simulink model "torqueBalancing"  (Simulink 8.6)
settings: Solver=FixedStepDiscrete  StartTime=0.0  StopTime=simulationTime  FixedStep=Ts  RelTol=1e-3
InitFcn:
  | initTorqueBalancing;
undefined symbols (not defined in the file): bVectorConstraints, ConstraintsMatrix, DEMO_MOVEMENTS, DiscIntNeverNeededParam, gain, impedencesSat, LEFT_RIGHT_FOOT_IN_CONTACT, localName, ON_GAZEBO, reg, ROBOT_DOF, ROBOT_DOF_FOR_SIMULINK, robotName, sat, sm, SMOOTH_DES_COM, SMOOTH_DES_Q, Ts, USE_QP_SOLVER, USE_SM
libraries: WBCLibrary x61, simulink x3
settings Model: Creator=daniele  LastModifiedBy=DanielePucci
settings DataIOCC: SignalLoggingSaveFormat=Dataset
settings DebuggingCC: FcnCallInpInsideContextMsg=EnableAllAsWarning
settings SFSimCC: SimParseCustomCode=off
settings ConfigComp: CovSFcnEnable=off

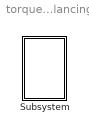
== system torqueBalancing ==
  Subsystem : Subsystem  mask{robotName=robotName, Ts=Ts, localName=localName}
      mask prompts: robotName "robot name"; localName "module name"

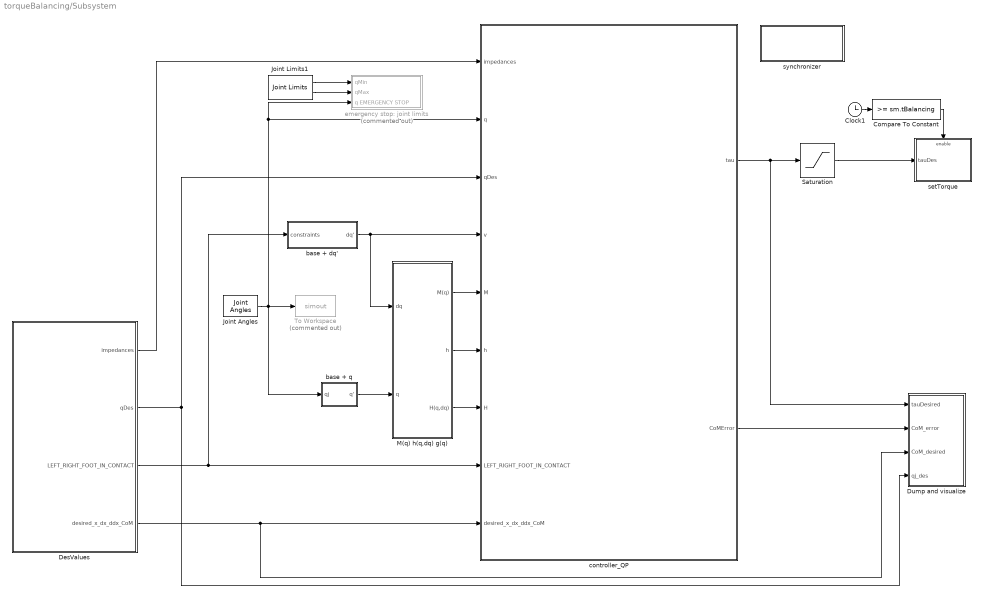
== system torqueBalancing/Subsystem ==
  Clock1 : Clock
  Compare To Constant : simulink/Logic and Bit Operations/Compare To Constant  relop=>=  const=sm.tBalancing  OutDataTypeStr=boolean
  DesValues : Subsystem  Priority=-10
  Dump and visualize : Subsystem
  Joint Angles : WBCLibrary/wholeBodyStates/Joint Angles  robotName=robotName  localName=localName
  Joint Limits1 : WBCLibrary/wholeBodyModel/Joint Limits  robotName=robotName  localName=localName
  M(q) h(q,dq) g(q) : Subsystem
  Saturation : Saturate  UpperLimit=sat.torque  LowerLimit=-sat.torque
  To Workspace : ToWorkspace  Commented=on  VariableName=simout  SaveFormat=Timeseries  SampleTime=-1
  base + dq' : Subsystem
  base + q : Subsystem
  controller_QP : Subsystem
  emergency stop: joint limits : Subsystem  Commented=on
  setTorque : Subsystem
  synchronizer : Subsystem
      mask Display: disp('SYNCHRONIZER')
  wires:
  base + q/1(q') -> M(q) h(q,dq) g(q)/2(q)
  base + dq'/1(dq') -> controller_QP/4(v), M(q) h(q,dq) g(q)/1(dq)
  M(q) h(q,dq) g(q)/1(M(q)) -> controller_QP/5(M)
  Joint Limits1/1 -> emergency stop: joint limits/1(qMin)
  Joint Limits1/2 -> emergency stop: joint limits/2(qMax)
  Joint Angles/1 -> To Workspace/1, base + q/1(qj), emergency stop: joint limits/3(q EMERGENCY STOP), controller_QP/2(q)
  M(q) h(q,dq) g(q)/2(h) -> controller_QP/6(h)
  M(q) h(q,dq) g(q)/3(H(q,dq)) -> controller_QP/7(H)
  controller_QP/1("tau ") -> Saturation/1, Dump and visualize/1(tauDesired)
  controller_QP/2(CoMError) -> Dump and visualize/2(CoM_error)
  DesValues/2(qDes) -> Dump and visualize/4(qj_des), controller_QP/3(qDes)
  DesValues/3(LEFT_RIGHT_FOOT_IN_CONTACT) -> base + dq'/1("constraints "), controller_QP/8(LEFT_RIGHT_FOOT_IN_CONTACT)
  DesValues/4(desired_x_dx_ddx_CoM) -> Dump and visualize/3(CoM_desired), controller_QP/9(desired_x_dx_ddx_CoM)
  DesValues/1(impedances) -> controller_QP/1(impedances)
  Saturation/1 -> setTorque/1(tauDes)
  Clock1/1 -> Compare To Constant/1
  Compare To Constant/1 -> setTorque/Enable

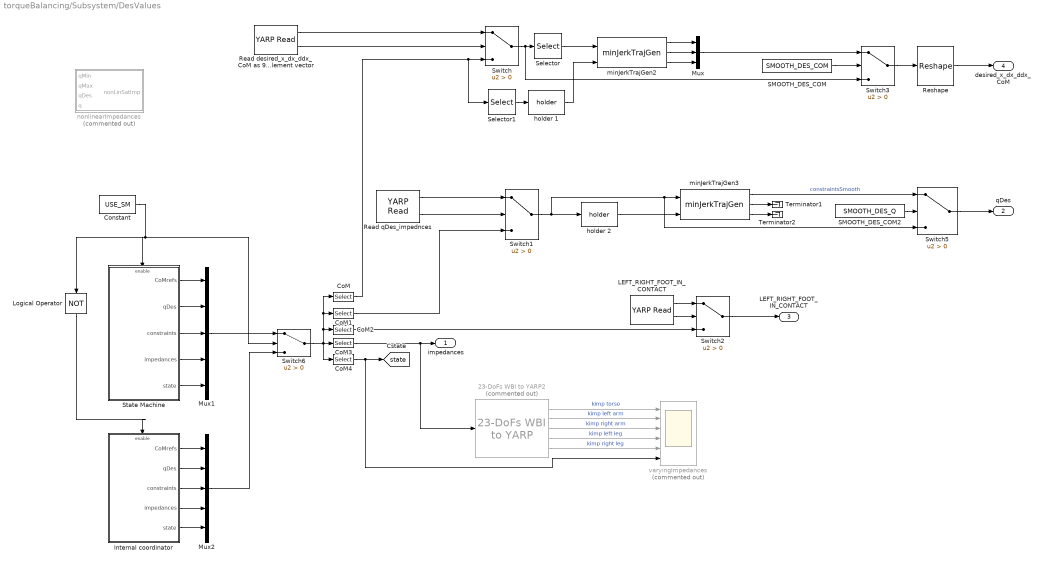
== system torqueBalancing/Subsystem/DesValues ==
  " LEFT_RIGHT_FOOT_IN_CONTACT" : WBCLibrary/Utilities/YARP Read  portName=['/' localName '/constraints:i']  signalSize=2  blocking=off  timestamp=off  autoconnect=off  errorOnConnection=on
  23-DoFs WBI to YARP2 : WBCLibrary/Utilities/23-DoFs WBI to YARP  Commented=on
  CoM : Selector  InputPortWidth=12+2*ROBOT_DOF  IndexOptions=Index vector (dialog)  Indices=[1:9]  OutputSizes=1
  CoM1 : Selector  InputPortWidth=12+2*ROBOT_DOF  IndexOptions=Index vector (dialog)  Indices=[10:9+ROBOT_DOF]  OutputSizes=1
  CoM2 : Selector  InputPortWidth=12+2*ROBOT_DOF  IndexOptions=Index vector (dialog)  Indices=[10+ROBOT_DOF,11+ROBOT_DOF]  OutputSizes=1
  CoM3 : Selector  InputPortWidth=12+2*ROBOT_DOF  IndexOptions=Index vector (dialog)  Indices=[12+ROBOT_DOF:11+2*ROBOT_DOF]  OutputSizes=1
  CoM4 : Selector  InputPortWidth=12+2*ROBOT_DOF  IndexOptions=Index vector (dialog)  Indices=[12+2*ROBOT_DOF]  OutputSizes=1
  Constant : Constant  Priority=-10  Value=USE_SM
  Internal coordinator : Subsystem
  Logical Operator : Logic  Operator=NOT  AllPortsSameDT=off  OutDataTypeStr=boolean
  Mux : Mux  Inputs=3
  Mux1 : Mux  Inputs=5
  Mux2 : Mux  Inputs=5
  "Read desired_x_dx_ddx_CoM as 9 element vector " : WBCLibrary/Utilities/YARP Read  portName=['/' localName '/comDes:i']  signalSize=9  blocking=off  timestamp=off  autoconnect=off  errorOnConnection=on
  Read qDes_impednces : WBCLibrary/Utilities/YARP Read  portName=['/' localName '/qDes:i']  signalSize=ROBOT_DOF  blocking=off  timestamp=off  autoconnect=off  errorOnConnection=on
  Reshape : Reshape  OutputDimensionality=Customize  OutputDimensions=[3,3]
  SMOOTH_DES_COM : Constant  Value=SMOOTH_DES_COM
  SMOOTH_DES_COM2 : Constant  Value=SMOOTH_DES_Q
  Selector : Selector  InputPortWidth=9  IndexOptions=Index vector (dialog)  Indices=[1 2 3]  OutputSizes=1
  Selector1 : Selector  InputPortWidth=9  IndexOptions=Index vector (dialog)  Indices=[1 2 3]  OutputSizes=1
  State Machine : Subsystem  Priority=-100
  Switch{,1..3,5..6} (6 alike) : Switch  Criteria=u2 > Threshold
  Terminator1 : Terminator
  Terminator2 : Terminator
  holder 1 : WBCLibrary/Utilities/holder 
  holder 2 : WBCLibrary/Utilities/holder 
  minJerkTrajGen2 : WBCLibrary/Utilities/minJerkTrajGen  dim=3  Ts=Ts  Tt=references.com.smoothingTime
  minJerkTrajGen3 : WBCLibrary/Utilities/minJerkTrajGen  dim=ROBOT_DOF  Ts=Ts  Tt=references.joints.smoothingTime
  nonlinearImpedances : Subsystem  Commented=on
  varyingImpedances : Scope  Commented=on  NumInputPorts=6
  impedances : Outport
  qDes : Outport  Port=2
  LEFT_RIGHT_FOOT_IN_CONTACT : Outport  Port=3
  desired_x_dx_ddx_CoM : Outport  Port=4
  tag scope: state=global
  wires:
  "Read desired_x_dx_ddx_CoM as 9 element vector "/2 -> Switch/2
  "Read desired_x_dx_ddx_CoM as 9 element vector "/1 -> Switch/1
  Reshape/1 -> desired_x_dx_ddx_CoM/1
  Read qDes_impednces/2 -> Switch1/2
  Read qDes_impednces/1 -> Switch1/1
  " LEFT_RIGHT_FOOT_IN_CONTACT"/2 -> Switch2/2
  " LEFT_RIGHT_FOOT_IN_CONTACT"/1 -> Switch2/1
  CoM2/1 -> Switch2/3
  CoM/1 -> Selector1/1, Switch/3
  CoM1/1 -> Switch1/3
  Switch/1 -> Switch3/3, Selector/1
  Selector/1 -> minJerkTrajGen2/1
  Selector1/1 -> holder 1/1
  holder 1/1 -> minJerkTrajGen2/2
  minJerkTrajGen2/1 -> Mux/1
  minJerkTrajGen2/2 -> Mux/2
  minJerkTrajGen2/3 -> Mux/3
  Mux/1 -> Switch3/1
  Switch3/1 -> Reshape/1
  SMOOTH_DES_COM/1 -> Switch3/2
  Switch2/1 -> LEFT_RIGHT_FOOT_IN_CONTACT/1
  minJerkTrajGen3/1 -> Switch5/1  "constraintsSmooth"
  SMOOTH_DES_COM2/1 -> Switch5/2
  Switch5/1 -> qDes/1
  Switch1/1 -> holder 2/1, Switch5/3, minJerkTrajGen3/1
  holder 2/1 -> minJerkTrajGen3/2
  minJerkTrajGen3/2 -> Terminator1/1
  minJerkTrajGen3/3 -> Terminator2/1
  Constant/1 -> Logical Operator/1, Switch6/2, State Machine/Enable
  Logical Operator/1 -> Internal coordinator/Enable
  State Machine/3(constraints) -> Mux1/3
  State Machine/2(qDes) -> Mux1/2
  State Machine/1(CoMrefs) -> Mux1/1
  Internal coordinator/1(CoMrefs) -> Mux2/1
  Internal coordinator/2(qDes) -> Mux2/2
  Internal coordinator/3(constraints) -> Mux2/3
  Mux2/1 -> Switch6/3
  Switch6/1 -> CoM4/1, CoM3/1, CoM/1, CoM1/1, CoM2/1
  Mux1/1 -> Switch6/1
  CoM3/1 -> 23-DoFs WBI to YARP2/1, impedances/1
  State Machine/4(impedances) -> Mux1/4
  Internal coordinator/4(impedances) -> Mux2/4
  23-DoFs WBI to YARP2/2 -> varyingImpedances/2  "kimp left arm"
  23-DoFs WBI to YARP2/4 -> varyingImpedances/4  "kimp left leg"
  23-DoFs WBI to YARP2/3 -> varyingImpedances/3  "kimp right arm"
  23-DoFs WBI to YARP2/5 -> varyingImpedances/5  "kimp right leg"
  23-DoFs WBI to YARP2/1 -> varyingImpedances/1  "kimp torso"
  State Machine/5(state) -> Mux1/5
  Internal coordinator/5(state) -> Mux2/5
  CoM4/1 -> varyingImpedances/6, [state]

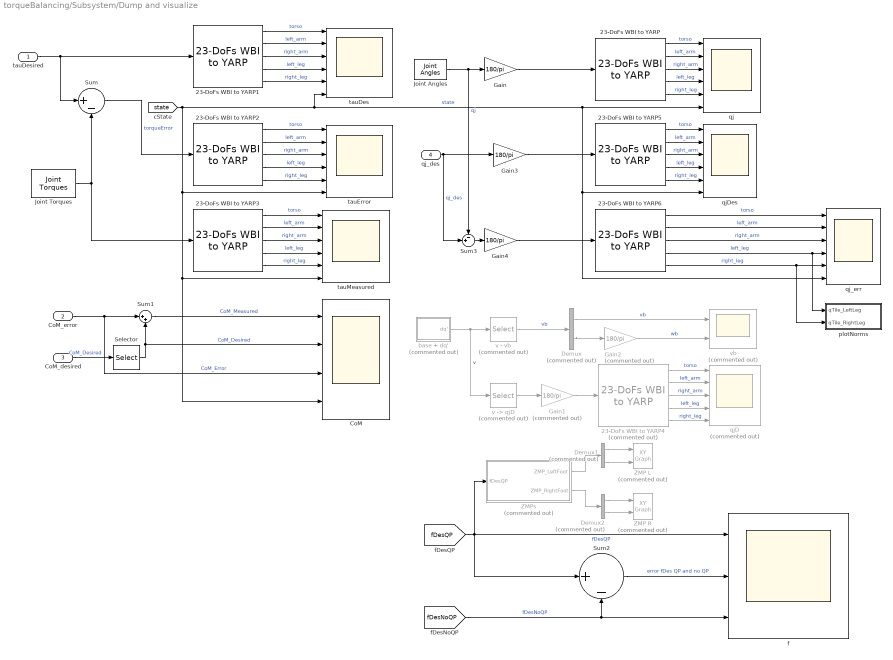
== system torqueBalancing/Subsystem/Dump and visualize ==
  tauDesired : Inport
  CoM_error : Inport  Port=2
  CoM_desired : Inport  Port=3
  qj_des : Inport  Port=4
  23-DoFs WBI to YARP{,1..3,5..6} (6 alike) : WBCLibrary/Utilities/23-DoFs WBI to YARP
  23-DoFs WBI to YARP4 : WBCLibrary/Utilities/23-DoFs WBI to YARP  Commented=on
  CoM : Scope  NumInputPorts=4
  Demux : Demux  Commented=on  Outputs=2
  Demux1 : Demux  Commented=on  Outputs=2
  Demux2 : Demux  Commented=on  Outputs=2
  Gain : Gain  Gain=180/pi
  Gain1 : Gain  Commented=on  Gain=180/pi
  Gain2 : Gain  Commented=on  Gain=180/pi
  Gain3 : Gain  Gain=180/pi
  Gain4 : Gain  Gain=180/pi
  Joint Angles : WBCLibrary/wholeBodyStates/Joint Angles  robotName=robotName  localName=localName
  Joint Torques : WBCLibrary/wholeBodyStates/Joint Torques  robotName=robotName  localName=localName
  Selector : Selector  NumberOfDimensions=2  IndexOptions=Index vector (dialog),Index vector (dialog)  Indices=[1:3],1  OutputSizes=1,1
  Sum : Sum  Inputs=|+-
  Sum1 : Sum  Inputs=|++
  Sum2 : Sum  Inputs=|+-
  Sum3 : Sum  Inputs=-+|
  ZMP L : simulink/Sinks/XY Graph  Commented=on  xmin=gain.footSize(1,1)  xmax=gain.footSize(1,2)  ymin=gain.footSize(2,1)  ymax=gain.footSize(2,2)  st=-1
  ZMP R : simulink/Sinks/XY Graph  Commented=on  xmin=gain.footSize(1,1)  xmax=gain.footSize(1,2)  ymin=gain.footSize(2,1)  ymax=gain.footSize(2,2)  st=-1
  ZMPs : Subsystem  Commented=on
  base + dq' : Subsystem  Commented=on
  f : Scope  NumInputPorts=3
  plotNorms : Subsystem
  qj : Scope  NumInputPorts=6
  qjD : Scope  Commented=on  NumInputPorts=5
  qjDes : Scope  NumInputPorts=6
  qj_err : Scope  NumInputPorts=6
  tauDes : Scope  NumInputPorts=6
  tauError : Scope  NumInputPorts=6
  tauMeasured : Scope  NumInputPorts=6
  v - vb : Selector  Commented=on  InputPortWidth=ROBOT_DOF+6  IndexOptions=Index vector (dialog)  Indices=[1:6]  OutputSizes=1
  "v -> qjD" : Selector  Commented=on  InputPortWidth=ROBOT_DOF+6  IndexOptions=Index vector (dialog)  Indices=[7:ROBOT_DOF+6]  OutputSizes=1
  vb : Scope  Commented=on  NumInputPorts=2
  wires:
  CoM_error/1 -> Sum1/1, CoM/3  "CoM_Error"
  CoM_desired/1 -> Selector/1  "CoM_Desired"
  Sum1/1 -> CoM/1  "CoM_Measured"
  base + dq'/1(dq') -> "v -> qjD"/1, v - vb/1  "v"
  Joint Angles/1 -> Sum3/1, Gain/1  "qj"
  Gain/1 -> 23-DoFs WBI to YARP/1
  23-DoFs WBI to YARP/5 -> qj/5  "right_leg"
  23-DoFs WBI to YARP/1 -> qj/1  "torso"
  23-DoFs WBI to YARP/2 -> qj/2  "left_arm"
  23-DoFs WBI to YARP/4 -> qj/4  "left_leg"
  23-DoFs WBI to YARP/3 -> qj/3  "right_arm"
  23-DoFs WBI to YARP4/5 -> qjD/5  "right_leg"
  23-DoFs WBI to YARP4/1 -> qjD/1  "torso"
  23-DoFs WBI to YARP4/2 -> qjD/2  "left_arm"
  23-DoFs WBI to YARP4/4 -> qjD/4  "left_leg"
  23-DoFs WBI to YARP4/3 -> qjD/3  "right_arm"
  "v -> qjD"/1 -> Gain1/1
  v - vb/1 -> Demux/1  "vb"
  Demux/1 -> vb/1  "vb"
  Demux/2 -> Gain2/1
  Gain1/1 -> 23-DoFs WBI to YARP4/1
  Gain2/1 -> vb/2  "wb"
  [fDesQP] -> ZMPs/1(fDesQP), Sum2/1, f/1  "fDesQP"
  ZMPs/1(ZMP_LeftFoot) -> Demux1/1
  ZMPs/2(ZMP_RightFoot) -> Demux2/1
  Demux1/1 -> ZMP L/1
  Demux1/2 -> ZMP L/2
  Demux2/1 -> ZMP R/1
  Demux2/2 -> ZMP R/2
  Sum2/1 -> f/2  "error fDes QP and no QP"
  [fDesNoQP] -> Sum2/2, f/3  "fDesNoQP"
  tauDesired/1 -> Sum/1, 23-DoFs WBI to YARP1/1
  Joint Torques/1 -> 23-DoFs WBI to YARP3/1, Sum/2
  23-DoFs WBI to YARP1/5 -> tauDes/5  "right_leg"
  23-DoFs WBI to YARP1/1 -> tauDes/1  "torso"
  23-DoFs WBI to YARP1/2 -> tauDes/2  "left_arm"
  23-DoFs WBI to YARP1/4 -> tauDes/4  "left_leg"
  23-DoFs WBI to YARP1/3 -> tauDes/3  "right_arm"
  23-DoFs WBI to YARP2/5 -> tauError/5  "right_leg"
  23-DoFs WBI to YARP2/1 -> tauError/1  "torso"
  23-DoFs WBI to YARP2/2 -> tauError/2  "left_arm"
  23-DoFs WBI to YARP2/4 -> tauError/4  "left_leg"
  23-DoFs WBI to YARP2/3 -> tauError/3  "right_arm"
  Sum/1 -> 23-DoFs WBI to YARP2/1  "torqueError"
  23-DoFs WBI to YARP3/5 -> tauMeasured/5  "right_leg"
  23-DoFs WBI to YARP3/1 -> tauMeasured/1  "torso"
  23-DoFs WBI to YARP3/2 -> tauMeasured/2  "left_arm"
  23-DoFs WBI to YARP3/4 -> tauMeasured/4  "left_leg"
  23-DoFs WBI to YARP3/3 -> tauMeasured/3  "right_arm"
  qj_des/1 -> Sum3/2, Gain3/1  "qj_des"
  Gain3/1 -> 23-DoFs WBI to YARP5/1
  23-DoFs WBI to YARP5/5 -> qjDes/5  "right_leg"
  23-DoFs WBI to YARP5/1 -> qjDes/1  "torso"
  23-DoFs WBI to YARP5/2 -> qjDes/2  "left_arm"
  23-DoFs WBI to YARP5/4 -> qjDes/4  "left_leg"
  23-DoFs WBI to YARP5/3 -> qjDes/3  "right_arm"
  Gain4/1 -> 23-DoFs WBI to YARP6/1
  23-DoFs WBI to YARP6/5 -> plotNorms/2(qTile_RightLeg), qj_err/5  "right_leg"
  23-DoFs WBI to YARP6/1 -> qj_err/1  "torso"
  23-DoFs WBI to YARP6/2 -> qj_err/2  "left_arm"
  23-DoFs WBI to YARP6/4 -> plotNorms/1(qTile_LeftLeg), qj_err/4  "left_leg"
  23-DoFs WBI to YARP6/3 -> qj_err/3  "right_arm"
  Sum3/1 -> Gain4/1
  Selector/1 -> Sum1/2, CoM/2  "CoM_Desired"
  [state] -> tauDes/6, qj_err/6, qjDes/6, qj/6, CoM/4, tauMeasured/6, tauError/6  "state"

== system torqueBalancing/Subsystem/M(q) h(q,dq) g(q) ==
  dq : Inport
  q : Inport  Port=2
  Cent Momentum : WBCLibrary/wholeBodyModel/Dynamics/Cent Momentum  robotName=robotName  localName=localName
  Gain : Gain  Commented=on  Gain=0
  computeh : WBCLibrary/wholeBodyModel/Dynamics/computeh  val=7  robotname=robotName  localname=localName
  computeh1 : WBCLibrary/wholeBodyModel/Dynamics/computeh  Commented=on  val=7  robotname=robotName  localname=localName
  massMatrix : WBCLibrary/wholeBodyModel/Dynamics/massMatrix  val=8  robotname=robotName  localname=localName
  M(q) : Outport
  h : Outport  Port=2
  H(q,dq) : Outport  Port=3
  wires:
  computeh/1 -> h/1
  massMatrix/1 -> M(q)/1
  q/1 -> computeh1/1, Cent Momentum/1, computeh/1, massMatrix/1
  dq/1 -> Gain/1, Cent Momentum/2, computeh/2
  Cent Momentum/1 -> H(q,dq)/1
  Gain/1 -> computeh1/2

== system torqueBalancing/Subsystem/base + dq' ==
  "constraints " : Inport
  Joint Velocities : WBCLibrary/wholeBodyStates/Joint Velocities  robotName=robotName  localName=localName
  Left Foot Jacobian : WBCLibrary/wholeBodyModel/Jacobians/Left Foot Jacobian  robotName=robotName  localName=localName
  MATLAB Function : MATLAB Function  TreatAsAtomicUnit=on
  Mux : Mux  Inputs=2
  Right Foot Jacobian : WBCLibrary/wholeBodyModel/Jacobians/Right Foot Jacobian  robotName=robotName  localName=localName
  dq' : Outport
  wires:
  Right Foot Jacobian/1 -> MATLAB Function/1(JcLeftFoot)
  Joint Velocities/1 -> MATLAB Function/4(qD), Mux/2
  Mux/1 -> dq'/1
  Left Foot Jacobian/1 -> MATLAB Function/2(JcRightFoot)
  "constraints "/1 -> MATLAB Function/3(activeFeetConstraints)
  MATLAB Function/1(y) -> Mux/1

== system torqueBalancing/Subsystem/base + q ==
  qj : Inport
  Constant1 : Constant  Value=zeros(16,1)
  Mux : Mux  Inputs=2
  q' : Outport
  wires:
  Mux/1 -> q'/1
  qj/1 -> Mux/2
  Constant1/1 -> Mux/1

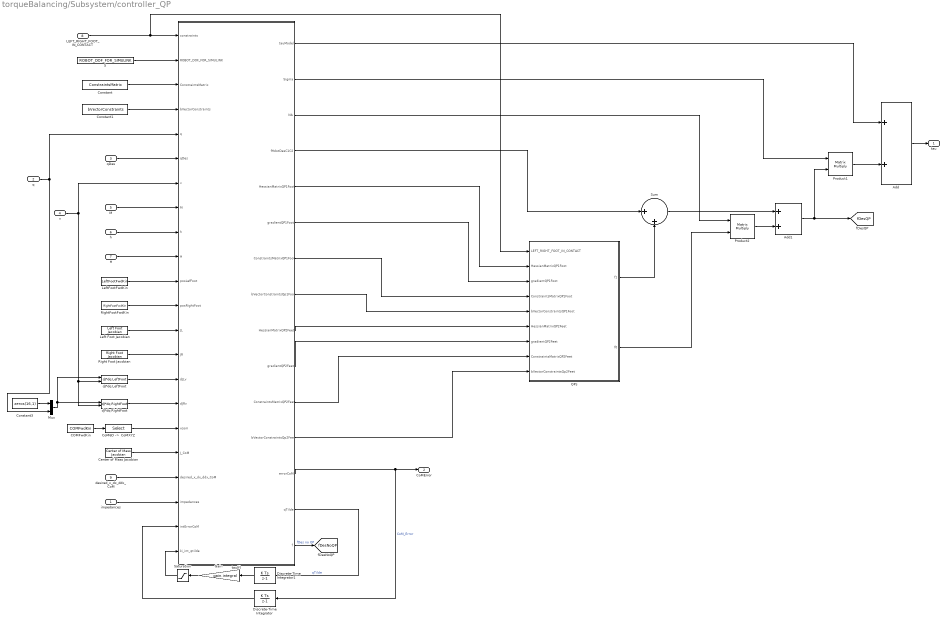
== system torqueBalancing/Subsystem/controller_QP ==
  impedances : Inport
  q : Inport  Port=2
  qDes : Inport  Port=3
  v : Inport  Port=4
  M : Inport  Port=5
  h : Inport  Port=6
  H : Inport  Port=7
  LEFT_RIGHT_FOOT_IN_CONTACT : Inport  Port=8
  desired_x_dx_ddx_CoM : Inport  Port=9
  "    5" : Constant  Value=ROBOT_DOF_FOR_SIMULINK
  Add : Sum
  Add1 : Sum
  "COMFwdKin " : WBCLibrary/wholeBodyModel/Forward Kinematics/COMFwdKin   robotName=robotName  localName=localName
  Center of Mass Jacobian : WBCLibrary/wholeBodyModel/Jacobians/Center of Mass Jacobian  robotName=robotName  localName=localName
  "CoM6D ->  CoMXYZ" : Selector  InputPortWidth=7  IndexOptions=Index vector (dialog)  Indices=[1 2 3]  OutputSizes=1
  Constant : Constant  Value=ConstraintsMatrix
  Constant1 : Constant  Value=bVectorConstraints
  Constant3 : Constant  Value=zeros(16,1)
  Discrete-Time Integrator : DiscreteIntegrator  InitialCondition=[0 0 0]  SampleTime=Ts  ICPrevOutput=DiscIntNeverNeededParam  ICPrevScaledInput=DiscIntNeverNeededParam
  Discrete-Time Integrator1 : DiscreteIntegrator  InitialCondition=zeros(ROBOT_DOF,1)  SampleTime=Ts  ICPrevOutput=DiscIntNeverNeededParam  ICPrevScaledInput=DiscIntNeverNeededParam
  Gain : Gain  Gain=gain.integral
  Left Foot Jacobian : WBCLibrary/wholeBodyModel/Jacobians/Left Foot Jacobian  robotName=robotName  localName=localName
  LeftFootFwdKin : WBCLibrary/wholeBodyModel/Forward Kinematics/LeftFootFwdKin  robotName=robotName  localName=localName
  Mux : Mux  Inputs=2
  Product1 : Product  Multiplication=Matrix(*)
  Product2 : Product  Multiplication=Matrix(*)
  QPs : Subsystem
  Right Foot Jacobian : WBCLibrary/wholeBodyModel/Jacobians/Right Foot Jacobian  robotName=robotName  localName=localName
  RightFootFwdKin : WBCLibrary/wholeBodyModel/Forward Kinematics/RightFootFwdKin  robotName=robotName  localName=localName
  Saturation : Saturate  UpperLimit=sat.integral  LowerLimit=-sat.integral
  Sum : Sum  Inputs=|++
  dJ*dq LeftFoot : WBCLibrary/wholeBodyModel/Dynamics/dJ*dq LeftFoot  val=9  robotName=robotName  localName=localName
  dJ*dq RightFoot : WBCLibrary/wholeBodyModel/Dynamics/dJ*dq RightFoot  val=9  robotName=robotName  localName=localName
  "tau(f) " : MATLAB Function  TreatAsAtomicUnit=on
  "tau " : Outport
  CoMError : Outport  Port=2
  tag scope: fDesNoQP=global, fDesQP=global
  wires:
  LEFT_RIGHT_FOOT_IN_CONTACT/1 -> QPs/1(LEFT_RIGHT_FOOT_IN_CONTACT), "tau(f) "/1(constraints)
  Discrete-Time Integrator/1 -> "tau(f) "/21(intErrorCoM)
  "tau(f) "/13(errorCoM) -> CoMError/1, Discrete-Time Integrator/1  "CoM_Error"
  Discrete-Time Integrator1/1 -> Gain/1
  "tau(f) "/14(qTilde) -> Discrete-Time Integrator1/1  "qTilde"
  Gain/1 -> Saturation/1
  Saturation/1 -> "tau(f) "/22(ki_int_qtilde)
  q/1 -> Mux/2, "tau(f) "/5(q)
  qDes/1 -> "tau(f) "/6(qDes)
  M/1 -> "tau(f) "/8(M)
  h/1 -> "tau(f) "/9(h)
  desired_x_dx_ddx_CoM/1 -> "tau(f) "/19(desired_x_dx_ddx_CoM)
  impedances/1 -> "tau(f) "/20(impedances)
  H/1 -> "tau(f) "/10(H)
  v/1 -> dJ*dq RightFoot/2, dJ*dq LeftFoot/2, "tau(f) "/7(v)
  Mux/1 -> dJ*dq LeftFoot/1, dJ*dq RightFoot/1
  "COMFwdKin "/1 -> "CoM6D ->  CoMXYZ"/1
  RightFootFwdKin/1 -> "tau(f) "/12(posRightFoot)
  LeftFootFwdKin/1 -> "tau(f) "/11(posLefFoot)
  Left Foot Jacobian/1 -> "tau(f) "/13(JL)
  Right Foot Jacobian/1 -> "tau(f) "/14(JR)
  dJ*dq LeftFoot/1 -> "tau(f) "/15(dJLv)
  Constant3/1 -> Mux/1
  dJ*dq RightFoot/1 -> "tau(f) "/16(dJRv)
  "CoM6D ->  CoMXYZ"/1 -> "tau(f) "/17(xcom)
  Center of Mass Jacobian/1 -> "tau(f) "/18(J_CoM)
  "tau(f) "/5(HessianMatrixQP1Foot) -> QPs/2(HessianMatrixQP1Foot)
  "tau(f) "/6(gradientQP1Foot) -> QPs/3(gradientQP1Foot)
  "tau(f) "/9(HessianMatrixQP2Feet) -> QPs/6(HessianMatrixQP2Feet)
  "tau(f) "/10(gradientQP2Feet) -> QPs/7(gradientQP2Feet)
  "tau(f) "/11(ConstraintsMatrixQP2Feet) -> QPs/8(ConstraintsMatrixQP2Feet)
  "tau(f) "/12(bVectorConstraintsQp2Feet) -> QPs/9(bVectorConstraintsQp2Feet)
  "tau(f) "/4(fHdotDesC1C2) -> Sum/1
  QPs/1(f1) -> Sum/2
  Product1/1 -> Add/2
  "tau(f) "/1(tauModel) -> Add/1
  Add/1 -> "tau "/1
  Add1/1 -> [fDesQP], Product1/2
  "    5"/1 -> "tau(f) "/2(ROBOT_DOF_FOR_SIMULINK)
  Constant/1 -> "tau(f) "/3(ConstraintsMatrix)
  Constant1/1 -> "tau(f) "/4(bVectorConstraints)
  "tau(f) "/7(ConstraintsMatrixQP1Foot) -> QPs/4(ConstraintsMatrixQP1Foot)
  "tau(f) "/8(bVectorConstraintsQp1Foot) -> QPs/5(bVectorConstraintsQP1Foot)
  Sum/1 -> Add1/1
  Product2/1 -> Add1/2
  "tau(f) "/3(NA) -> Product2/1
  QPs/2(f0) -> Product2/2
  "tau(f) "/2(Sigma) -> Product1/1
  "tau(f) "/15(f) -> [fDesNoQP]  "fDes no QP"

== system torqueBalancing/Subsystem/emergency stop: joint limits ==
  qMin : Inport
  qMax : Inport  Port=2
  q EMERGENCY STOP : Inport  Port=3
  Assertion : Assertion
  MATLAB Function : MATLAB Function  TreatAsAtomicUnit=on
  index1 : Constant  Value=0.01  VectorParams1D=off
  wires:
  qMin/1 -> MATLAB Function/1(umin)
  qMax/1 -> MATLAB Function/2(umax)
  index1/1 -> MATLAB Function/4(tol)
  q EMERGENCY STOP/1 -> MATLAB Function/3(u)
  MATLAB Function/1(inRange) -> Assertion/1

== system torqueBalancing/Subsystem/setTorque ==
  tauDes : Inport
  Enable : EnablePort
  Set Torques1 : WBCLibrary/wholeBodyActuators/Set Torques  val=6  robotName=robotName  localName=localName
  wires:
  tauDes/1 -> Set Torques1/1

== system torqueBalancing/Subsystem/synchronizer ==
  GAZEBO_SYNCHRONIZER : Subsystem  Commented=on
  Logical Operator : Logic  Operator=NOT  AllPortsSameDT=off  OutDataTypeStr=boolean
  "ON_GAZEBO " : Constant  Value=ON_GAZEBO
  REAL_TIME_SYNC : Subsystem
  wires:
  Logical Operator/1 -> REAL_TIME_SYNC/Enable
  "ON_GAZEBO "/1 -> GAZEBO_SYNCHRONIZER/Enable, Logical Operator/1

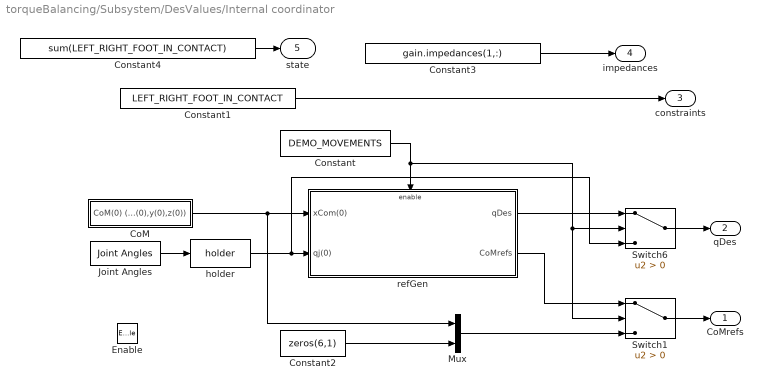
== system torqueBalancing/Subsystem/DesValues/Internal coordinator ==
  Enable : EnablePort
  "CoM " : Subsystem
  Constant : Constant  Value=DEMO_MOVEMENTS
  Constant1 : Constant  Value=LEFT_RIGHT_FOOT_IN_CONTACT
  Constant2 : Constant  Value=zeros(6,1)
  Constant3 : Constant  Value=gain.impedances(1,:)
  Constant4 : Constant  Value=sum(LEFT_RIGHT_FOOT_IN_CONTACT)
  Joint Angles : WBCLibrary/wholeBodyStates/Joint Angles  robotName=robotName  localName=localName
  Mux : Mux  Inputs=2
  Switch1 : Switch  Criteria=u2 > Threshold
  Switch6 : Switch  Criteria=u2 > Threshold
  "holder " : WBCLibrary/Utilities/holder 
  refGen : Subsystem
  CoMrefs : Outport
  qDes : Outport  Port=2
  constraints : Outport  Port=3
  impedances : Outport  Port=4
  state : Outport  Port=5
  wires:
  Constant1/1 -> constraints/1
  Joint Angles/1 -> "holder "/1
  "CoM "/1(CoM(0) (x(0),y(0),z(0))) -> Mux/1, refGen/1(xCom(0))
  "holder "/1 -> Switch6/3, refGen/2(qj(0))
  Constant/1 -> Switch1/2, Switch6/2, refGen/Enable
  Switch6/1 -> qDes/1
  Switch1/1 -> CoMrefs/1
  refGen/1(qDes) -> Switch6/1
  refGen/2(CoMrefs) -> Switch1/1
  Mux/1 -> Switch1/3
  Constant2/1 -> Mux/2
  Constant3/1 -> impedances/1
  Constant4/1 -> state/1

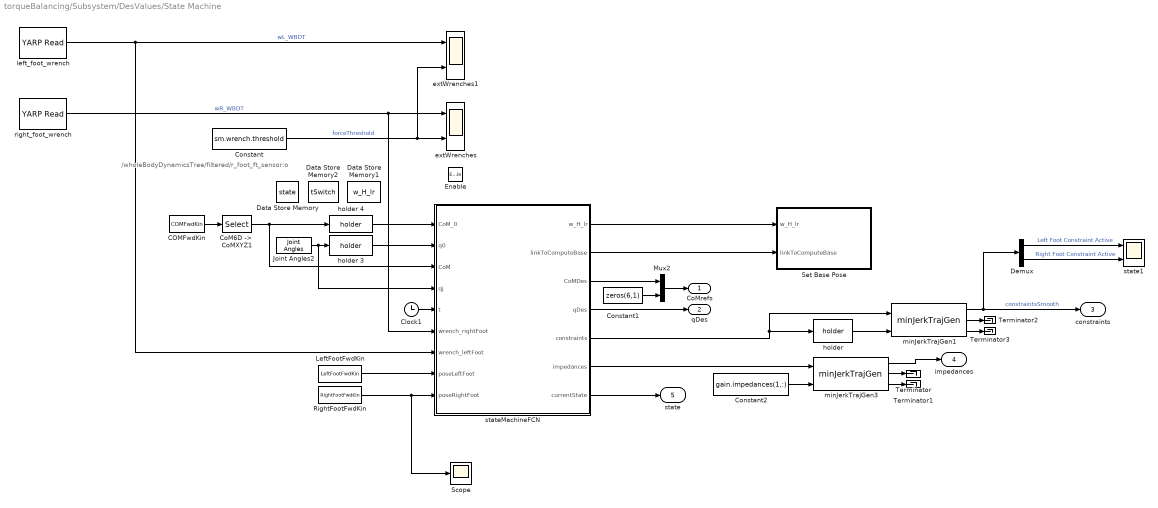
== system torqueBalancing/Subsystem/DesValues/State Machine ==
  note: /wholeBodyDynamicsTree/filtered/r_foot_ft_sensor:o
  Enable : EnablePort
  "COMFwdKin " : WBCLibrary/wholeBodyModel/Forward Kinematics/COMFwdKin   robotName=robotName  localName=localName
  Clock1 : Clock
  "CoM6D ->  CoMXYZ1" : Selector  InputPortWidth=7  IndexOptions=Index vector (dialog)  Indices=[1 2 3]  OutputSizes=1
  Constant : Constant  Value=sm.wrench.threshold
  Constant1 : Constant  Value=zeros(6,1)
  Constant2 : Constant  Value=gain.impedances(1,:)
  Data Store Memory : DataStoreMemory  DataStoreName=state  InitialValue=sm.stateAt0  OutDataTypeStr=double
  Data Store Memory1 : DataStoreMemory  DataStoreName=w_H_lr  InitialValue=eye(4)  OutDataTypeStr=double
  Data Store Memory2 : DataStoreMemory  DataStoreName=tSwitch  OutDataTypeStr=double
  Demux : Demux  Outputs=2
  Joint Angles2 : WBCLibrary/wholeBodyStates/Joint Angles  robotName=robotName  localName=localName
  LeftFootFwdKin : WBCLibrary/wholeBodyModel/Forward Kinematics/LeftFootFwdKin  robotName=robotName  localName=localName
  Mux2 : Mux  Inputs=2
  RightFootFwdKin : WBCLibrary/wholeBodyModel/Forward Kinematics/RightFootFwdKin  robotName=robotName  localName=localName
  Scope : Scope
  Set Base Pose : Subsystem
  Terminator{,1..3} (4 alike) : Terminator
  extWrenches : Scope  NumInputPorts=2
  extWrenches1 : Scope  NumInputPorts=2
  "holder " : WBCLibrary/Utilities/holder 
  holder 3 : WBCLibrary/Utilities/holder 
  holder 4 : WBCLibrary/Utilities/holder 
  left_foot_wrench : WBCLibrary/Utilities/YARP Read  portName='/wholeBodyDynamicsTree/left_leg/cartesianEndEffectorWrench:o'  signalSize=6  blocking=off  timestamp=off  autoconnect=on  errorOnConnection=off
  minJerkTrajGen1 : WBCLibrary/Utilities/minJerkTrajGen  dim=2  Ts=Ts  Tt=smoothingTimeTransitionDynamics
  minJerkTrajGen3 : WBCLibrary/Utilities/minJerkTrajGen  dim=ROBOT_DOF  Ts=Ts  Tt=gain.SmoothingTimeImp
  right_foot_wrench : WBCLibrary/Utilities/YARP Read  portName='/wholeBodyDynamicsTree/right_leg/cartesianEndEffectorWrench:o'  signalSize=6  blocking=off  timestamp=off  autoconnect=on  errorOnConnection=off
  state1 : Scope  NumInputPorts=2
  stateMachineFCN : MATLAB Function  TreatAsAtomicUnit=on
  CoMrefs : Outport
  qDes : Outport  Port=2
  constraints : Outport  Port=3
  impedances : Outport  Port=4
  state : Outport  Port=5
  wires:
  Constant/1 -> extWrenches1/2, extWrenches/2  "forceThreshold"
  right_foot_wrench/1 -> extWrenches/1, stateMachineFCN/6(wrench_rightFoot)  "wR_WBDT"
  Joint Angles2/1 -> stateMachineFCN/4(qj), holder 3/1
  "COMFwdKin "/1 -> "CoM6D ->  CoMXYZ1"/1
  "CoM6D ->  CoMXYZ1"/1 -> stateMachineFCN/3(CoM), holder 4/1
  holder 4/1 -> stateMachineFCN/1(CoM_0)
  holder 3/1 -> stateMachineFCN/2(q0)
  Clock1/1 -> stateMachineFCN/5(t)
  stateMachineFCN/4(qDes) -> qDes/1
  stateMachineFCN/3(CoMDes) -> Mux2/1
  Mux2/1 -> CoMrefs/1
  Constant1/1 -> Mux2/2
  stateMachineFCN/6(impedances) -> minJerkTrajGen3/1
  Constant2/1 -> minJerkTrajGen3/2
  minJerkTrajGen3/1 -> impedances/1
  minJerkTrajGen3/2 -> Terminator/1
  minJerkTrajGen3/3 -> Terminator1/1
  stateMachineFCN/7(currentState) -> state/1
  minJerkTrajGen1/1 -> Demux/1, constraints/1  "constraintsSmooth"
  minJerkTrajGen1/2 -> Terminator2/1
  minJerkTrajGen1/3 -> Terminator3/1
  stateMachineFCN/5(constraints) -> minJerkTrajGen1/1, "holder "/1
  Demux/1 -> state1/1  "Left Foot Constraint Active"
  Demux/2 -> state1/2  "Right Foot Constraint Active"
  "holder "/1 -> minJerkTrajGen1/2
  LeftFootFwdKin/1 -> stateMachineFCN/8(poseLeftFoot)
  RightFootFwdKin/1 -> Scope/1, stateMachineFCN/9(poseRightFoot)
  left_foot_wrench/1 -> extWrenches1/1, stateMachineFCN/7(wrench_leftFoot)  "wL_WBDT"
  stateMachineFCN/2(linkToComputeBase) -> Set Base Pose/2(linkToComputeBase)
  stateMachineFCN/1(w_H_lr) -> Set Base Pose/1(w_H_lr)

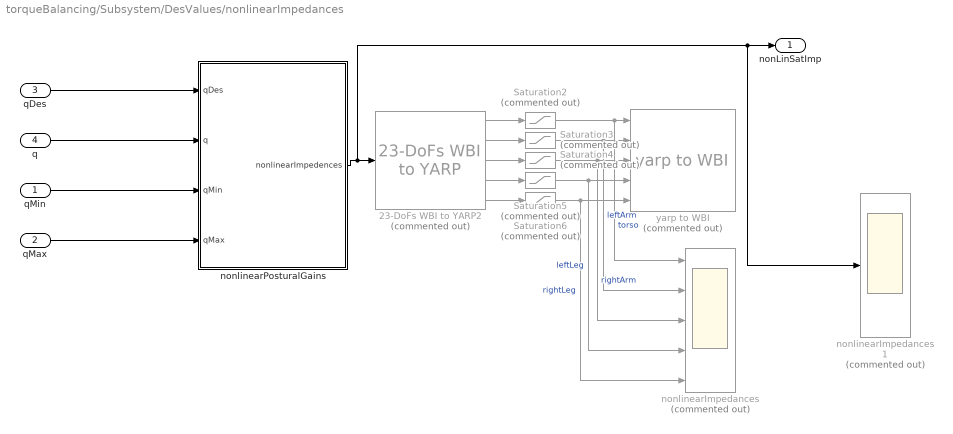
== system torqueBalancing/Subsystem/DesValues/nonlinearImpedances ==
  qMin : Inport
  qMax : Inport  Port=2
  qDes : Inport  Port=3
  q : Inport  Port=4
  23-DoFs WBI to YARP2 : WBCLibrary/Utilities/23-DoFs WBI to YARP  Commented=on
  Saturation2 : Saturate  Commented=on  UpperLimit=impedencesSat(1)  LowerLimit=0  SampleTime=Ts
  Saturation3 : Saturate  Commented=on  UpperLimit=impedencesSat(2)  LowerLimit=0  SampleTime=Ts
  Saturation4 : Saturate  Commented=on  UpperLimit=impedencesSat(2)  LowerLimit=0  SampleTime=Ts
  Saturation5 : Saturate  Commented=on  UpperLimit=impedencesSat(3)  LowerLimit=0  SampleTime=Ts
  Saturation6 : Saturate  Commented=on  UpperLimit=impedencesSat(3)  LowerLimit=0  SampleTime=Ts
  nonlinearImpedances : Scope  Commented=on  NumInputPorts=5
  nonlinearImpedances1 : Scope  Commented=on
  "nonlinearPosturalGains " : MATLAB Function  TreatAsAtomicUnit=on
  yarp to WBI : WBCLibrary/Utilities/yarp to WBI  Commented=on
  nonLinSatImp : Outport
  wires:
  23-DoFs WBI to YARP2/1 -> Saturation2/1
  23-DoFs WBI to YARP2/2 -> Saturation3/1
  23-DoFs WBI to YARP2/3 -> Saturation4/1
  23-DoFs WBI to YARP2/5 -> Saturation6/1
  "nonlinearPosturalGains "/1(nonlinearImpedences) -> nonlinearImpedances1/1, nonLinSatImp/1, 23-DoFs WBI to YARP2/1
  qMin/1 -> "nonlinearPosturalGains "/3(qMin)
  qMax/1 -> "nonlinearPosturalGains "/4(qMax)
  q/1 -> "nonlinearPosturalGains "/2(q)
  Saturation6/1 -> nonlinearImpedances/5, yarp to WBI/5  "rightLeg"
  Saturation4/1 -> nonlinearImpedances/3, yarp to WBI/3  "rightArm"
  Saturation5/1 -> nonlinearImpedances/4, yarp to WBI/4  "leftLeg"
  Saturation3/1 -> nonlinearImpedances/2, yarp to WBI/2  "leftArm"
  Saturation2/1 -> nonlinearImpedances/1, yarp to WBI/1  "torso"
  23-DoFs WBI to YARP2/4 -> Saturation5/1
  qDes/1 -> "nonlinearPosturalGains "/1(qDes)

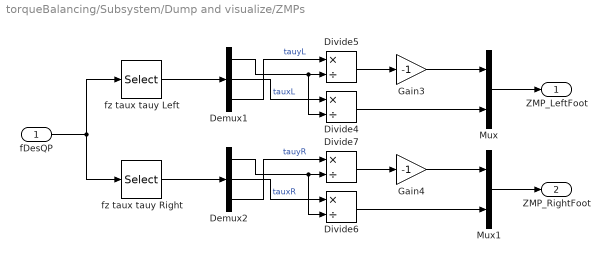
== system torqueBalancing/Subsystem/Dump and visualize/ZMPs ==
  fDesQP : Inport
  Demux1 : Demux  Outputs=3
  Demux2 : Demux  Outputs=3
  Divide{4..7} (4 alike) : Product  Inputs=*/
  Gain3 : Gain  Gain=-1
  Gain4 : Gain  Gain=-1
  Mux : Mux  Inputs=2
  Mux1 : Mux  Inputs=2
  fz taux tauy Left : Selector  InputPortWidth=12  IndexOptions=Index vector (dialog)  Indices=[3 4 5]  OutputSizes=1
  fz taux tauy Right : Selector  InputPortWidth=12  IndexOptions=Index vector (dialog)  Indices=[9 10 11]  OutputSizes=1
  ZMP_LeftFoot : Outport
  ZMP_RightFoot : Outport  Port=2
  wires:
  fz taux tauy Left/1 -> Demux1/1
  Demux1/1 -> Divide4/2, Divide5/2
  Divide7/1 -> Gain4/1
  Divide4/1 -> Mux/2
  Divide5/1 -> Gain3/1
  fz taux tauy Right/1 -> Demux2/1
  Demux2/1 -> Divide6/2, Divide7/2
  fDesQP/1 -> fz taux tauy Left/1, fz taux tauy Right/1
  Gain3/1 -> Mux/1
  Mux/1 -> ZMP_LeftFoot/1
  Divide6/1 -> Mux1/2
  Gain4/1 -> Mux1/1
  Mux1/1 -> ZMP_RightFoot/1
  Demux1/2 -> Divide4/1  "tauxL"
  Demux1/3 -> Divide5/1  "tauyL"
  Demux2/2 -> Divide6/1  "tauxR"
  Demux2/3 -> Divide7/1  "tauyR"

== system torqueBalancing/Subsystem/Dump and visualize/base + dq' ==
  Joint Velocities : WBCLibrary/wholeBodyStates/Joint Velocities  robotName=robotName  localName=localName
  Left Foot Jacobian : WBCLibrary/wholeBodyModel/Jacobians/Left Foot Jacobian  robotName=robotName  localName=localName
  Mux : Mux  Inputs=2
  Right Foot Jacobian : WBCLibrary/wholeBodyModel/Jacobians/Right Foot Jacobian  robotName=robotName  localName=localName
  baseVelocity : Subsystem  AncestorBlock=WBCLibrary/Utilities/baseVelocity  mask(baseVelocity){}
      mask help: This block computes the velocity of the floating base of a bipedal robot
  dq' : Outport
  wires:
  Left Foot Jacobian/1 -> baseVelocity/2(JacobLF)
  Right Foot Jacobian/1 -> baseVelocity/1(JacobRF)
  baseVelocity/1(baseVel) -> Mux/1
  Joint Velocities/1 -> baseVelocity/3(dq), Mux/2
  Mux/1 -> dq'/1

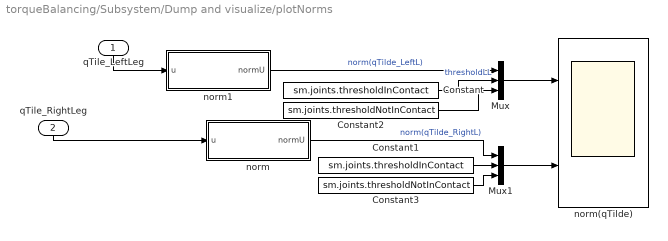
== system torqueBalancing/Subsystem/Dump and visualize/plotNorms ==
  qTile_LeftLeg : Inport
  qTile_RightLeg : Inport  Port=2
  Constant : Constant  Value=sm.joints.thresholdInContact
  Constant1 : Constant  Value=sm.joints.thresholdInContact
  Constant2 : Constant  Value=sm.joints.thresholdNotInContact
  Constant3 : Constant  Value=sm.joints.thresholdNotInContact
  Mux : Mux  Inputs=3
  Mux1 : Mux  Inputs=3
  norm : MATLAB Function  TreatAsAtomicUnit=on
  norm(qTilde) : Scope  NumInputPorts=2
  norm1 : MATLAB Function  TreatAsAtomicUnit=on
  wires:
  Constant/1 -> Mux/2  "thresholdLL"
  qTile_LeftLeg/1 -> norm1/1(u)
  qTile_RightLeg/1 -> norm/1(u)
  norm/1(normU) -> Mux1/1  "norm(qTilde_RightL)"
  norm1/1(normU) -> Mux/1  "norm(qTilde_LeftL)"
  Mux/1 -> norm(qTilde)/1
  Mux1/1 -> norm(qTilde)/2
  Constant2/1 -> Mux/3
  Constant1/1 -> Mux1/2
  Constant3/1 -> Mux1/3

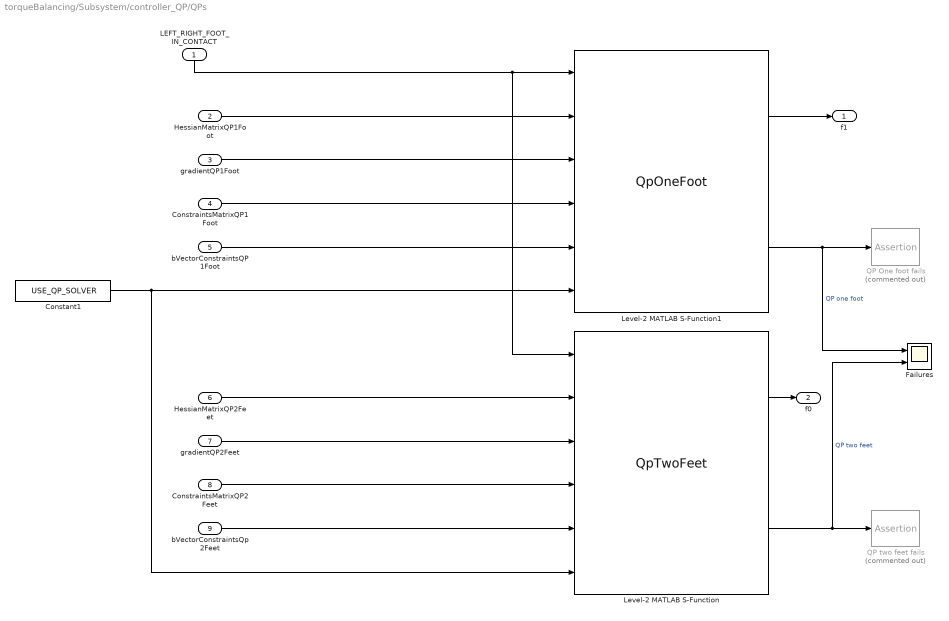
== system torqueBalancing/Subsystem/controller_QP/QPs ==
  LEFT_RIGHT_FOOT_IN_CONTACT : Inport
  HessianMatrixQP1Foot : Inport  Port=2
  gradientQP1Foot : Inport  Port=3
  ConstraintsMatrixQP1Foot : Inport  Port=4
  bVectorConstraintsQP1Foot : Inport  Port=5
  HessianMatrixQP2Feet : Inport  Port=6
  gradientQP2Feet : Inport  Port=7
  ConstraintsMatrixQP2Feet : Inport  Port=8
  bVectorConstraintsQp2Feet : Inport  Port=9
  Constant1 : Constant  Value=USE_QP_SOLVER
  Failures : Scope  NumInputPorts=2
  Level-2 MATLAB S-Function : M-S-Function  FunctionName=QpTwoFeet
  Level-2 MATLAB S-Function1 : M-S-Function  FunctionName=QpOneFoot
  QP One foot fails : Assertion  Commented=on
  QP two feet fails : Assertion  Commented=on
  f1 : Outport
  f0 : Outport  Port=2
  wires:
  LEFT_RIGHT_FOOT_IN_CONTACT/1 -> Level-2 MATLAB S-Function/1, Level-2 MATLAB S-Function1/1
  gradientQP2Feet/1 -> Level-2 MATLAB S-Function/3
  HessianMatrixQP1Foot/1 -> Level-2 MATLAB S-Function1/2
  ConstraintsMatrixQP2Feet/1 -> Level-2 MATLAB S-Function/4
  gradientQP1Foot/1 -> Level-2 MATLAB S-Function1/3
  HessianMatrixQP2Feet/1 -> Level-2 MATLAB S-Function/2
  Level-2 MATLAB S-Function/1 -> f0/1
  bVectorConstraintsQp2Feet/1 -> Level-2 MATLAB S-Function/5
  Level-2 MATLAB S-Function1/1 -> f1/1
  ConstraintsMatrixQP1Foot/1 -> Level-2 MATLAB S-Function1/4
  bVectorConstraintsQP1Foot/1 -> Level-2 MATLAB S-Function1/5
  Level-2 MATLAB S-Function/2 -> Failures/2, QP two feet fails/1  "QP two feet"
  Constant1/1 -> Level-2 MATLAB S-Function/6, Level-2 MATLAB S-Function1/6
  Level-2 MATLAB S-Function1/2 -> Failures/1, QP One foot fails/1  "QP one foot"

== system torqueBalancing/Subsystem/synchronizer/GAZEBO_SYNCHRONIZER ==
  Enable : EnablePort
  synchronize : WBCLibrary/Utilities/synchronize  rate=0.010  scaleFactor=1

== system torqueBalancing/Subsystem/synchronizer/REAL_TIME_SYNC ==
  Enable : EnablePort
  Real Time Synchronizer : WBCLibrary/Utilities/Real Time Synchronizer  threadPeriod=Ts

== system torqueBalancing/Subsystem/DesValues/Internal coordinator/CoM  ==
  "COMFwdKin " : WBCLibrary/wholeBodyModel/Forward Kinematics/COMFwdKin   robotName=robotName  localName=localName
  "CoM6D ->  CoMXYZ" : Selector  InputPortWidth=7  IndexOptions=Index vector (dialog)  Indices=[1 2 3]  OutputSizes=1
  "holder " : WBCLibrary/Utilities/holder 
  CoM(0) (x(0),y(0),z(0)) : Outport
  wires:
  "COMFwdKin "/1 -> "CoM6D ->  CoMXYZ"/1
  "CoM6D ->  CoMXYZ"/1 -> "holder "/1
  "holder "/1 -> CoM(0) (x(0),y(0),z(0))/1

== system torqueBalancing/Subsystem/DesValues/Internal coordinator/refGen ==
  xCom(0) : Inport
  qj(0) : Inport  Port=2
  Enable : EnablePort
  Clock1 : Clock
  refGenFCN : MATLAB Function  TreatAsAtomicUnit=on
  qDes : Outport
  CoMrefs : Outport  Port=2
  wires:
  refGenFCN/2(desired_x_dx_ddx_CoM) -> CoMrefs/1
  xCom(0)/1 -> refGenFCN/1(xCom0)
  Clock1/1 -> refGenFCN/3(t)
  qj(0)/1 -> refGenFCN/2(q0)
  refGenFCN/1(qDes) -> qDes/1

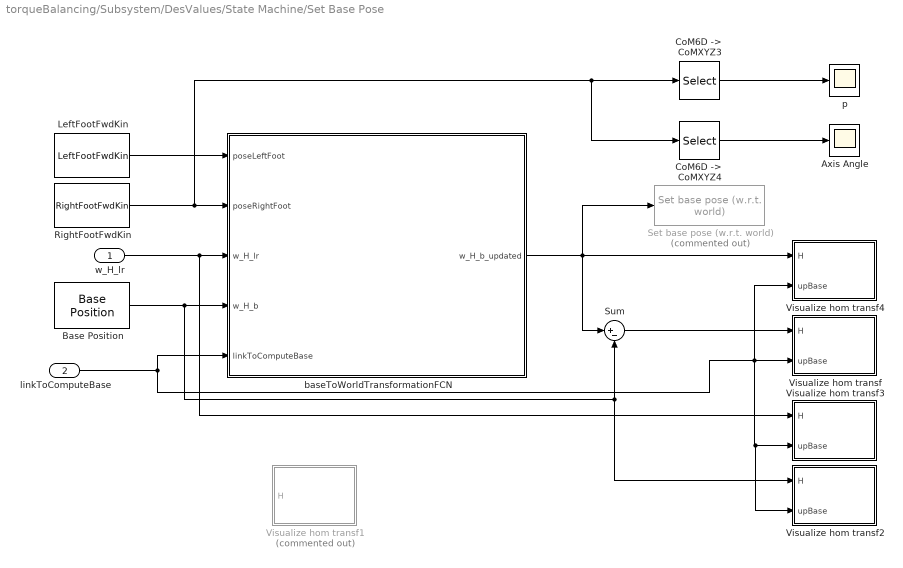
== system torqueBalancing/Subsystem/DesValues/State Machine/Set Base Pose ==
  w_H_lr : Inport
  linkToComputeBase : Inport  Port=2
  Axis Angle : Scope
  Base Position : WBCLibrary/wholeBodyStates/Base Position  robotName=robotName  localName=localName
  "CoM6D ->  CoMXYZ3" : Selector  InputPortWidth=7  IndexOptions=Index vector (dialog)  Indices=[1 2 3]  OutputSizes=1
  "CoM6D ->  CoMXYZ4" : Selector  InputPortWidth=7  IndexOptions=Index vector (dialog)  Indices=[4 5 6 7]  OutputSizes=1
  LeftFootFwdKin : WBCLibrary/wholeBodyModel/Forward Kinematics/LeftFootFwdKin  robotName=robotName  localName=localName
  RightFootFwdKin : WBCLibrary/wholeBodyModel/Forward Kinematics/RightFootFwdKin  robotName=robotName  localName=localName
  Set base pose (w.r.t. world) : WBCLibrary/wholeBodyStates/Set base pose (w.r.t. world)  Commented=on
  Sum : Sum  Inputs=|+-
  Visualize hom transf : Subsystem
  Visualize hom transf1 : Subsystem  Commented=on
  Visualize hom transf2 : Subsystem
  Visualize hom transf3 : Subsystem
  Visualize hom transf4 : Subsystem
  baseToWorldTransformationFCN : MATLAB Function  Priority=-20  TreatAsAtomicUnit=on
  p : Scope
  wires:
  baseToWorldTransformationFCN/1(w_H_b_updated) -> Set base pose (w.r.t. world)/1, Sum/1, Visualize hom transf4/1(H)
  "CoM6D ->  CoMXYZ3"/1 -> p/1
  w_H_lr/1 -> Visualize hom transf3/1(H), baseToWorldTransformationFCN/3(w_H_lr)
  Base Position/1 -> Visualize hom transf2/1(H), Sum/2, baseToWorldTransformationFCN/4(w_H_b)
  Sum/1 -> Visualize hom transf/1(H)
  linkToComputeBase/1 -> baseToWorldTransformationFCN/5(linkToComputeBase), Visualize hom transf2/2(upBase), Visualize hom transf3/2(upBase), Visualize hom transf4/2(upBase), Visualize hom transf/2(upBase)
  RightFootFwdKin/1 -> "CoM6D ->  CoMXYZ4"/1, "CoM6D ->  CoMXYZ3"/1, baseToWorldTransformationFCN/2(poseRightFoot)
  "CoM6D ->  CoMXYZ4"/1 -> Axis Angle/1
  LeftFootFwdKin/1 -> baseToWorldTransformationFCN/1(poseLeftFoot)

== system torqueBalancing/Subsystem/Dump and visualize/base + dq'/baseVelocity ==
  JacobRF : Inport
  JacobLF : Inport  Port=2
  dq : Inport  Port=3
  Constant : Constant  Value=LEFT_RIGHT_FOOT_IN_CONTACT
  MATLAB Function : MATLAB Function  TreatAsAtomicUnit=on
  baseVel : Outport
  wires:
  JacobLF/1 -> MATLAB Function/1(JcLeftFoot)
  JacobRF/1 -> MATLAB Function/2(JcRightFoot)
  MATLAB Function/1(y) -> baseVel/1
  dq/1 -> MATLAB Function/4(qD)
  Constant/1 -> MATLAB Function/3(activeFeetConstraints)

== system torqueBalancing/Subsystem/DesValues/State Machine/Set Base Pose/Visualize hom transf ==
  H : Inport
  upBase : Inport  Port=2
  "CoM6D ->  CoMXYZ1" : Selector  NumberOfDimensions=2  InputPortWidth=7  IndexOptions=Index vector (dialog),Index vector (dialog)  Indices=[1 2 3],[1 2 3]  OutputSizes=1,1
  "CoM6D ->  CoMXYZ2" : Selector  NumberOfDimensions=2  InputPortWidth=7  IndexOptions=Index vector (dialog),Index vector (dialog)  Indices=[1 2 3],[4]  OutputSizes=1,1
  Hom : Scope  NumInputPorts=2
  R : Scope  NumInputPorts=2
  p : Scope  NumInputPorts=2
  wires:
  "CoM6D ->  CoMXYZ1"/1 -> R/1
  "CoM6D ->  CoMXYZ2"/1 -> p/1
  H/1 -> "CoM6D ->  CoMXYZ2"/1, Hom/1, "CoM6D ->  CoMXYZ1"/1
  upBase/1 -> p/2, R/2, Hom/2

== system torqueBalancing/Subsystem/DesValues/State Machine/Set Base Pose/Visualize hom transf1 ==
  H : Inport
  "CoM6D ->  CoMXYZ1" : Selector  NumberOfDimensions=2  InputPortWidth=7  IndexOptions=Index vector (dialog),Index vector (dialog)  Indices=[1 2 3],[1 2 3]  OutputSizes=1,1
  "CoM6D ->  CoMXYZ2" : Selector  NumberOfDimensions=2  InputPortWidth=7  IndexOptions=Index vector (dialog),Index vector (dialog)  Indices=[1 2 3],[4]  OutputSizes=1,1
  Hom : Scope
  R : Scope
  p : Scope
  wires:
  "CoM6D ->  CoMXYZ1"/1 -> R/1
  "CoM6D ->  CoMXYZ2"/1 -> p/1
  H/1 -> "CoM6D ->  CoMXYZ2"/1, Hom/1, "CoM6D ->  CoMXYZ1"/1

== system torqueBalancing/Subsystem/DesValues/State Machine/Set Base Pose/Visualize hom transf2 ==
  H : Inport
  upBase : Inport  Port=2
  "CoM6D ->  CoMXYZ1" : Selector  NumberOfDimensions=2  InputPortWidth=7  IndexOptions=Index vector (dialog),Index vector (dialog)  Indices=[1 2 3],[1 2 3]  OutputSizes=1,1
  "CoM6D ->  CoMXYZ2" : Selector  NumberOfDimensions=2  InputPortWidth=7  IndexOptions=Index vector (dialog),Index vector (dialog)  Indices=[1 2 3],[4]  OutputSizes=1,1
  Hom : Scope  NumInputPorts=2
  R : Scope  NumInputPorts=2
  p : Scope  NumInputPorts=2
  wires:
  "CoM6D ->  CoMXYZ1"/1 -> R/1
  "CoM6D ->  CoMXYZ2"/1 -> p/1
  H/1 -> "CoM6D ->  CoMXYZ2"/1, Hom/1, "CoM6D ->  CoMXYZ1"/1
  upBase/1 -> p/2, R/2, Hom/2

== system torqueBalancing/Subsystem/DesValues/State Machine/Set Base Pose/Visualize hom transf3 ==
  H : Inport
  upBase : Inport  Port=2
  "CoM6D ->  CoMXYZ1" : Selector  NumberOfDimensions=2  InputPortWidth=7  IndexOptions=Index vector (dialog),Index vector (dialog)  Indices=[1 2 3],[1 2 3]  OutputSizes=1,1
  "CoM6D ->  CoMXYZ2" : Selector  NumberOfDimensions=2  InputPortWidth=7  IndexOptions=Index vector (dialog),Index vector (dialog)  Indices=[1 2 3],[4]  OutputSizes=1,1
  Hom : Scope  NumInputPorts=2
  R : Scope  NumInputPorts=2
  p : Scope  NumInputPorts=2
  wires:
  "CoM6D ->  CoMXYZ1"/1 -> R/1
  "CoM6D ->  CoMXYZ2"/1 -> p/1
  H/1 -> "CoM6D ->  CoMXYZ2"/1, Hom/1, "CoM6D ->  CoMXYZ1"/1
  upBase/1 -> p/2, R/2, Hom/2

== system torqueBalancing/Subsystem/DesValues/State Machine/Set Base Pose/Visualize hom transf4 ==
  H : Inport
  upBase : Inport  Port=2
  "CoM6D ->  CoMXYZ1" : Selector  NumberOfDimensions=2  InputPortWidth=7  IndexOptions=Index vector (dialog),Index vector (dialog)  Indices=[1 2 3],[1 2 3]  OutputSizes=1,1
  "CoM6D ->  CoMXYZ2" : Selector  NumberOfDimensions=2  InputPortWidth=7  IndexOptions=Index vector (dialog),Index vector (dialog)  Indices=[1 2 3],[4]  OutputSizes=1,1
  Hom : Scope  NumInputPorts=2
  R : Scope  NumInputPorts=2
  p : Scope  NumInputPorts=2
  wires:
  "CoM6D ->  CoMXYZ1"/1 -> R/1
  "CoM6D ->  CoMXYZ2"/1 -> p/1
  H/1 -> "CoM6D ->  CoMXYZ2"/1, Hom/1, "CoM6D ->  CoMXYZ1"/1
  upBase/1 -> p/2, R/2, Hom/2

== matlab function Subsystem/DesValues/Internal coordinator/refGen/refGenFCN ==
  data: xCom0 input double; qDes output double; q0 input double; t input double; references parameter double; desired_x_dx_ddx_CoM output double
function [qDes,desired_x_dx_ddx_CoM] = refGenFCN(xCom0,q0,t,references)
%#codegen

[qDes,desired_x_dx_ddx_CoM] = refGen(xCom0,q0,t,references);

== matlab function Subsystem/base + dq'/MATLAB Function ==
  data: JcLeftFoot input double; JcRightFoot input double; activeFeetConstraints input double; y output double; qD input double; reg parameter double
function y = fcn(JcLeftFoot,JcRightFoot,activeFeetConstraints,qD,reg)
%#codegen

Jc = [activeFeetConstraints(1)*JcLeftFoot;
      activeFeetConstraints(2)*JcRightFoot];

pinvJb = (Jc(:,1:6)'*Jc(:,1:6) + reg.pinvDampVb*eye(6))\Jc(:,1:6)';  
  
% pinvJb = pinv(Jc(:,1:6));

y = -pinvJb*Jc(:,7:end)*qD;

== matlab function Subsystem/emergency stop: joint limits/MATLAB Function ==
  data: umin input double; umax input double; u input double; inRange output double; tol input double
function inRange = checkRange(umin, umax, u, tol)
%#codegen

res = u < umin + tol | u > umax - tol;
res = sum(res);
if res==0
    inRange = 1;
else
    inRange = 0;
    u < umin + tol | u > umax - tol
end

== matlab function Subsystem/controller_QP/tau(f)  ==
  data: tauModel output double; Sigma output double; NA output double; fHdotDesC1C2 output double; HessianMatrixQP1Foot output double; gradientQP1Foot output double; ConstraintsMatrixQP1Foot output double; bVectorConstraintsQp1Foot output double; HessianMatrixQP2Feet output double; gradientQP2Feet output double; ConstraintsMatrixQP2Feet output double; bVectorConstraintsQp2Feet output double; constraints input double; ROBOT_DOF_FOR_SIMULINK input double; ConstraintsMatrix input double; bVectorConstraints input double; q input double; qDes input double; v input double; M input double; h input double; H input double; posLefFoot input double; posRightFoot input double; JL input double; JR input double; dJLv input double; dJRv input double; xcom input double; J_CoM input double; desired_x_dx_ddx_CoM input double; impedances input double; intErrorCoM input double; ki_int_qtilde input double; reg parameter double; gain parameter double; errorCoM output double; qTilde output double; f output double
function [tauModel,Sigma,NA,fHdotDesC1C2, ...
          HessianMatrixQP1Foot,gradientQP1Foot,ConstraintsMatrixQP1Foot,bVectorConstraintsQp1Foot,...
          HessianMatrixQP2Feet,gradientQP2Feet,ConstraintsMatrixQP2Feet,bVectorConstraintsQp2Feet,...
          errorCoM,qTilde,f]    =  ...
          controllerFCN(constraints,ROBOT_DOF_FOR_SIMULINK,ConstraintsMatrix,bVectorConstraints,...
          q,qDes,v, M, h , H, posLefFoot, posRightFoot, JL,JR, dJLv,dJRv, xcom,J_CoM, desired_x_dx_ddx_CoM,...
          impedances, intErrorCoM,ki_int_qtilde,reg,gain)
%#codegen

footSize       = gain.footSize;
gainsPCOM      = gain.PCOM;
gainsICOM      = gain.ICOM;
gainsDCOM      = gain.DCOM;
gainMomentum   = gain.PAngularMomentum;
dampings       = gain.dampings;

e1              = [1;0;0];
e2              = [0;1;0];
e3              = [0;0;1]; 
ROBOT_DOF       = size(ROBOT_DOF_FOR_SIMULINK,1);


gravAcc         = 9.81;
m               = M(1,1);
Mb              = M(1:6,1:6);
Mbj             = M(1:6,7:end);
% Mj              = M(7:end,7:end);

St              = [  zeros(6,ROBOT_DOF);
                   eye(ROBOT_DOF,ROBOT_DOF)];
grav            = [ zeros(2,1);
                   -m*gravAcc;
                    zeros(3,1)];
                
pos_leftFoot   = posLefFoot(1:3);
rotMatLeftFoot = Rf(posLefFoot(4:7));

pos_rightFoot   = posRightFoot(1:3);
rotMatRightFoot = Rf(posRightFoot(4:7));


xDcom           = J_CoM(1:3,:)*v;
qD              = v(7:end);
xDDcomStar      = desired_x_dx_ddx_CoM(:,3) - gainsPCOM*(xcom - desired_x_dx_ddx_CoM(:,1)) - gainsICOM*intErrorCoM - gainsDCOM*(xDcom - desired_x_dx_ddx_CoM(:,2));
Pr              = pos_rightFoot - xcom; % Application point of the contact force on the right foot w.r.t. CoM
Pl              = pos_leftFoot  - xcom; % Application point of the contact force on the left foot w.r.t. CoM


AL = [ eye(3),   zeros(3);
       Sf(Pl),  eye(3)];
AR = [ eye(3), zeros(3);
        Sf(Pr), eye(3) ];
    
A    = [ AL, AR];

Jc   = [ JL*constraints(1) ;
         JR*constraints(2)];
JcDv = [ dJLv*constraints(1) ;
         dJRv*constraints(2)];

JcMinv          = Jc/M;
JcMinvSt        = JcMinv*St;
JcMinvJct       = JcMinv*transpose(Jc);

pinvA         = pinv( A, reg.pinvTol)*constraints(1)*constraints(2) + [inv(AL);zeros(6)]*constraints(1)*(1-constraints(2)) + [zeros(6);inv(AR)]*constraints(2)*(1-constraints(1)); 
% PInv_JcMinvSt = pinv( JcMinvSt, PINV_TOL);
PInv_JcMinvSt = JcMinvSt'/(JcMinvSt*JcMinvSt' + reg.pinvDamp*eye(size(JcMinvSt,1)));
  
HDotDes  = [ m*xDDcomStar ;
            -gainMomentum*H(4:end)]; 
         

NL        = eye(ROBOT_DOF) - PInv_JcMinvSt*JcMinvSt;

f_HDot           = pinvA*(HDotDes - grav);

fHdotDesC1C2     =  f_HDot*constraints(1)*constraints(2);

NA               = (eye(12,12)-pinvA*A)*constraints(1)*constraints(2);
JBar             = transpose(Jc(:,7:end)) - Mbj'/Mb*transpose(Jc(:,1:6)); % multiplier of f in tau0

qTilde           =  q-qDes;


Sigma            = -(PInv_JcMinvSt*JcMinvJct + NL*JBar);
SigmaNA          = Sigma*NA;

tauModel         = PInv_JcMinvSt*(JcMinv*h - JcDv) + NL*(h(7:end) - Mbj'/Mb*h(1:6) - diag(impedances)*qTilde  -ki_int_qtilde -diag(dampings)*NL*qD);

CL               = ConstraintsMatrix; 
CL(end-4,1:3)    = -e3'*rotMatLeftFoot;                
CL(end-3,:)      = [ footSize(1,1)*e3'*rotMatLeftFoot', e2'*rotMatLeftFoot'];
CL(end-2,:)      = [-footSize(1,2)*e3'*rotMatLeftFoot',-e2'*rotMatLeftFoot'];

CL(end-1,:)      = [ footSize(2,1)*e3'*rotMatLeftFoot',-e1'*rotMatLeftFoot'];
CL(end  ,:)      = [-footSize(2,2)*e3'*rotMatLeftFoot', e1'*rotMatLeftFoot'];

CR               = ConstraintsMatrix;
CR(end-4,1:3)    = -e3'*rotMatRightFoot;  
CR(end-3,:)      = [ footSize(1,1)*e3'*rotMatRightFoot', e2'*rotMatRightFoot'];
CR(end-2,:)      = [-footSize(1,2)*e3'*rotMatRightFoot',-e2'*rotMatRightFoot'];

CR(end-1,:)      = [ footSize(2,1)*e3'*rotMatRightFoot',-e1'*rotMatRightFoot'];
CR(end  ,:)      = [-footSize(2,2)*e3'*rotMatRightFoot', e1'*rotMatRightFoot'];


ConstraintsMatrix2Feet   = blkdiag(CL,CR);
bVectorConstraints2Feet  = [bVectorConstraints;bVectorConstraints];

ConstraintsMatrixQP1Foot = constraints(1) * (1 - constraints(2)) * CL + ...
                           constraints(2) * (1 - constraints(1)) * CR;
bVectorConstraintsQp1Foot= bVectorConstraints;

ConstraintsMatrixQP2Feet  = ConstraintsMatrix2Feet*NA;
bVectorConstraintsQp2Feet = bVectorConstraints2Feet-ConstraintsMatrix2Feet*f_HDot;

HessianMatrixQP2Feet      = SigmaNA'*SigmaNA + eye(size(SigmaNA,2))*reg.HessianQP;
gradientQP2Feet           = SigmaNA'*(tauModel + Sigma*f_HDot);

A1Foot                    = AL*constraints(1)*(1-constraints(2)) + AR*constraints(2)*(1-constraints(1));
HessianMatrixQP1Foot      = A1Foot'*A1Foot + eye(size(A1Foot,2))*reg.HessianQP;
gradientQP1Foot           = -A1Foot'*(HDotDes - grav);

f0                        = -pinv(SigmaNA, reg.pinvTol)*(tauModel + Sigma*f_HDot);

f                         = f_HDot + NA*f0;

errorCoM = xcom - desired_x_dx_ddx_CoM(:,1);

== matlab function Subsystem/Dump and visualize/plotNorms/norm ==
  data: u input double; normU output double
function normU = fcn(u)
%#codegen

normU = norm(u);

== matlab function Subsystem/Dump and visualize/base + dq'/baseVelocity/MATLAB Function ==
  data: JcLeftFoot input double; JcRightFoot input double; activeFeetConstraints input double; y output double; qD input double
function y = fcn(JcLeftFoot,JcRightFoot,activeFeetConstraints,qD)
%#codegen
if sum(activeFeetConstraints) == 2
    Jc = [JcLeftFoot;JcRightFoot];
else
    Jc = JcLeftFoot;
end
y = -pinv(Jc(:,1:6))*Jc(:,7:end)*qD;

== matlab function Subsystem/DesValues/nonlinearImpedances/nonlinearPosturalGains  ==
  data: qDes input double; nonlinearImpedences output double; q input double; qMin input double; qMax input double; gain parameter double
function nonlinearImpedences = fcn(qDes,q,qMin,qMax,gain)
    %#codegen
    impedences_at_0     = gain.impedances;
    increasingRatesImp  = (gain.increasingRatesImp)';
    qTildeMax           = gain.qTildeMax;

    tp =  pi./(2*(qMax-qDes));
    tn = -pi./(2*(qMin-qDes));

    
    qTilde = q - qDes;
            
    nonlinearImpedences = (impedences_at_0'   + increasingRatesImp.*tan(pi.*qTilde./(2*qTildeMax)).^2)';
%                                                increasingRatesImp.*tan((tp.*stepFcn(qTilde) + tn.*stepFcn(-qTilde)).*qTilde).^2)';
                                           
end

function y = stepFcn(x) 
   %#codegen
   y = x > 0; 
end

== matlab function Subsystem/Dump and visualize/plotNorms/norm1 ==
  data: u input double; normU output double
function normU = fcn(u)
%#codegen

normU = norm(u);

== matlab function Subsystem/DesValues/State Machine/Set Base Pose/baseToWorldTransformationFCN ==
  data: poseLeftFoot input double; poseRightFoot input double; w_H_lr input double; w_H_b input double; linkToComputeBase input double; w_H_b_updated output double
function w_H_b_updated = baseToWorldTransformationFCN(poseLeftFoot,poseRightFoot,w_H_lr,w_H_b,linkToComputeBase)
%#codegen

    w_H_b_updated = baseToWorldTransformation(poseLeftFoot,poseRightFoot,w_H_lr,w_H_b,linkToComputeBase);
    
end

== matlab function Subsystem/DesValues/State Machine/stateMachineFCN ==
  data: w_H_lr output double; linkToComputeBase output double; CoMDes output double; qDes output double; constraints output double; state data_store_memory double; CoM_0 input double; q0 input double; CoM input double; qj input double; t input double; wrench_rightFoot input double; wrench_leftFoot input double; poseLeftFoot input double; poseRightFoot input double; tSwitch data_store_memory double; sm parameter double; impedances output double; gain parameter double; currentState output double
function [w_H_lr,linkToComputeBase, CoMDes,qDes,constraints,impedances,currentState] = stateMachineFCN(CoM_0, q0, CoM,qj, t, wrench_rightFoot,wrench_leftFoot,poseLeftFoot,poseRightFoot, sm,gain)
%#codegen

[CoMDes,qDes,constraints, currentState,impedances,w_H_lr,linkToComputeBase] = stateMachine(CoM_0, q0, CoM,qj, t, wrench_rightFoot,wrench_leftFoot,poseLeftFoot,poseRightFoot, sm,gain);
